simulink model "Lab2"  (R2016a)
settings: Solver=VariableStepAuto  StartTime=0.0  StopTime=10.0  RelTol=1e-3
libraries: simulink x3, dspsigops x1
settings Model: Creator=DELL  LastModifiedBy=DELL

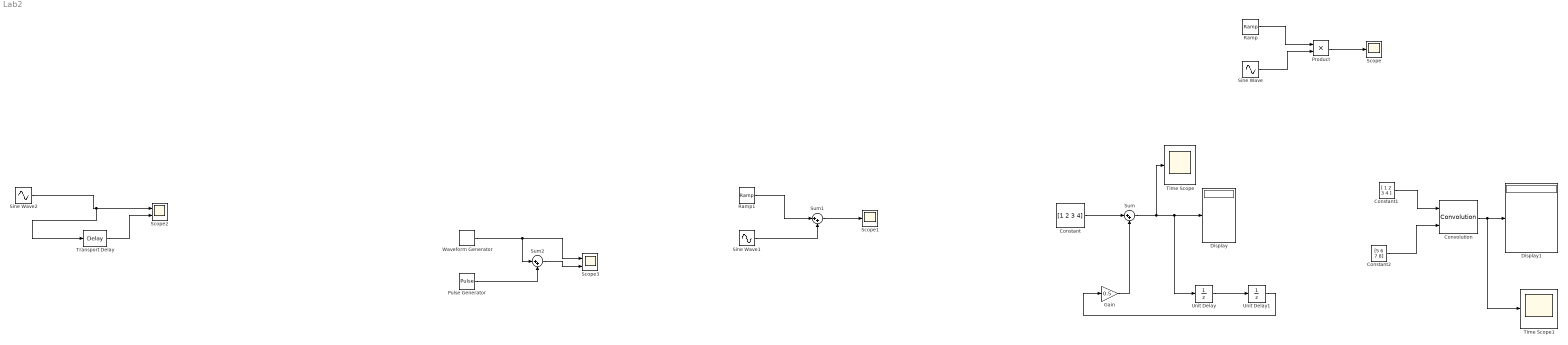
== system Lab2 ==
  Constant : Constant  Value=[1 2 3 4]  SampleTime=1e-1
  Constant1 : Constant  Value=[ 1 2 3 4 ]  SampleTime=1e-1
  Constant2 : Constant  Value=[5 6 7 8]  SampleTime=1e-1
  Convolution : dspsigops/Convolution  domain=Time  outputDataTypeStr=Inherit: Same as accumulator  outputLastDataTypeStr=Inherit: Same as accumulator  outputMin=[]  outputMax=[]  roundingMode=Floor  overflowMode=off
  Display : Display
  Display1 : Display
  Gain : Gain  Gain=0.5
  Product : Product
  Pulse Generator : DiscretePulseGenerator  PulseType=Time based  Period=10  PulseWidth=5
  Ramp : simulink/Sources/Ramp  slope=1  start=0  X0=0
  Ramp1 : simulink/Sources/Ramp  slope=1  start=0  X0=0
  Scope : Scope
  Scope1 : Scope
  Scope2 : Scope  NumInputPorts=2
  Scope3 : Scope  NumInputPorts=2
  Sine Wave : Sin  SampleTime=0
  Sine Wave1 : Sin  SampleTime=0
  Sine Wave2 : Sin  SampleTime=0
  Sum : Sum  Inputs=|++
  Sum1 : Sum  Inputs=|++
  Sum2 : Sum  Inputs=|++
  Time Scope : Scope
  Time Scope1 : Scope
  Transport Delay : TransportDelay
  Unit Delay : UnitDelay  SampleTime=-1
  Unit Delay1 : UnitDelay  SampleTime=-1
  Waveform Generator : simulink/Sources/Waveform Generator  OutMin=[]  OutMax=[]  OutDataTypeStr=double  SelectedSignal=1  BlockNames=MultiportSwitch_e3df3653d217406  SampleTime=0.1
  wires:
  Constant/1 -> Sum/1
  Sum/1 -> Time Scope/1, Unit Delay/1, Display/1
  Gain/1 -> Sum/2
  Unit Delay/1 -> Unit Delay1/1
  Unit Delay1/1 -> Gain/1
  Constant1/1 -> Convolution/1
  Constant2/1 -> Convolution/2
  Convolution/1 -> Time Scope1/1, Display1/1
  Ramp/1 -> Product/1
  Sine Wave/1 -> Product/2
  Product/1 -> Scope/1
  Sum1/1 -> Scope1/1
  Sine Wave1/1 -> Sum1/2
  Ramp1/1 -> Sum1/1
  Transport Delay/1 -> Scope2/2
  Sine Wave2/1 -> Transport Delay/1, Scope2/1
  Pulse Generator/1 -> Sum2/2
  Waveform Generator/1 -> Sum2/1, Scope3/1
  Sum2/1 -> Scope3/2
